simulink model "msd"  (R2013a)
settings: Solver=ode45  StartTime=0.0  StopTime=10.0  RelTol=1e-3
settings Model: Creator=yak  LastModifiedBy=yak

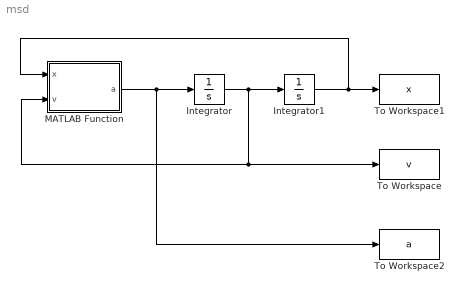
== system msd ==
  Integrator : Integrator
  Integrator1 : Integrator  InitialCondition=-5
  MATLAB Function : MATLAB Function  TreatAsAtomicUnit=on
  To Workspace : ToWorkspace  VariableName=v  SampleTime=-1  SaveFormat=Timeseries
  To Workspace1 : ToWorkspace  VariableName=x  SampleTime=-1  SaveFormat=Timeseries
  To Workspace2 : ToWorkspace  VariableName=a  SampleTime=-1  SaveFormat=Timeseries
  wires:
  Integrator1/1 -> MATLAB Function/1(x), To Workspace1/1
  Integrator/1 -> MATLAB Function/2(v), To Workspace/1, Integrator1/1
  MATLAB Function/1(a) -> To Workspace2/1, Integrator/1

== matlab function msd/MATLAB Function ==
  data: x input; a output; v input
function a = dyn(x, v)
%#codegen

a = -(0.5*v + 5*x)/1;
